simulink model "FloatingBall"  (R2024b)
settings: Solver=FixedStepAuto  StartTime=0.0  StopTime=inf  RelTol=1e-3  EnableMultiTasking=on
undefined symbols (not defined in the file or in its folder): Start
libraries: arduinolib x10, arduinoavrlib x2
(part 1 of 2)
settings Model: ExtModeTrigDuration=2  Creator=Tim  LastModifiedBy=thoma
settings SolverCC: AutoInsertRateTranBlk=on
settings OptimizationCC: DefaultParameterBehavior=Inlined  EnhancedBackFolding=on  PassReuseOutputArgsAs=Individual arguments  ZeroExternalMemoryAtStartup=off  ZeroInternalMemoryAtStartup=off  MaxStackSize=64  OptimizeBlockOrder=speed  DifferentSizesBufferReuse=on  OptimizationCustomize=off  EfficientTunableParamExpr=on
settings DebuggingCC: MultiTaskDSMMsg=none  ParameterTunabilityLossMsg=error
settings HardwareCC: ProdBitPerInt=16  ProdBitPerPointer=16  ProdBitPerSizeT=16  ProdBitPerPtrDiffT=16  ProdLargestAtomicFloat=None  ProdWordSize=8  ProdHWDeviceType=Atmel->AVR
settings SFSimCC: MATLABDynamicMemAlloc=off
settings RTWCC: Description=Embedded Coder  SystemTargetFile=ert.tlc  HardwareBoard=Arduino Uno  TemplateMakefile=ert_default_tmf  Toolchain=Arduino AVR  BuildConfiguration=Faster Runs
settings CodeAppCC: ForceParamTrailComments=on  IgnoreCustomStorageClasses=off  OperatorAnnotations=on  SimulinkDataObjDesc=on  SFDataObjDesc=on  InsertBlockDesc=on
settings ERTTargetCC: SupportContinuousTime=on  SupportVariableSizeSignals=on  ExtModeTransport=3  ExtModeStaticAlloc=on  ExtModeAutomaticAllocSize=off  ExtModeStaticAllocSize=250  ExtModeMexFile=ext_xcp  ExtModeIntrfLevel=Level2 - Open

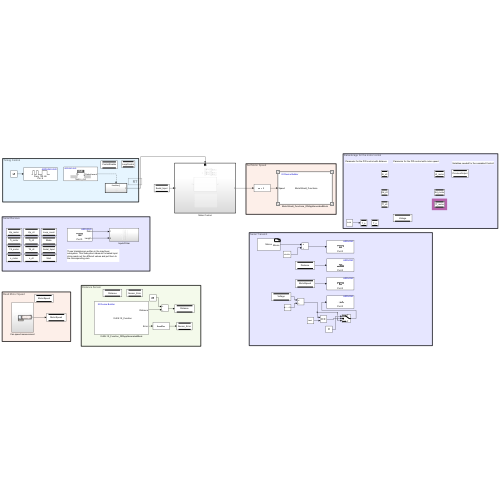
[thumbnail: Simulink's stored preview of the top-level diagram]
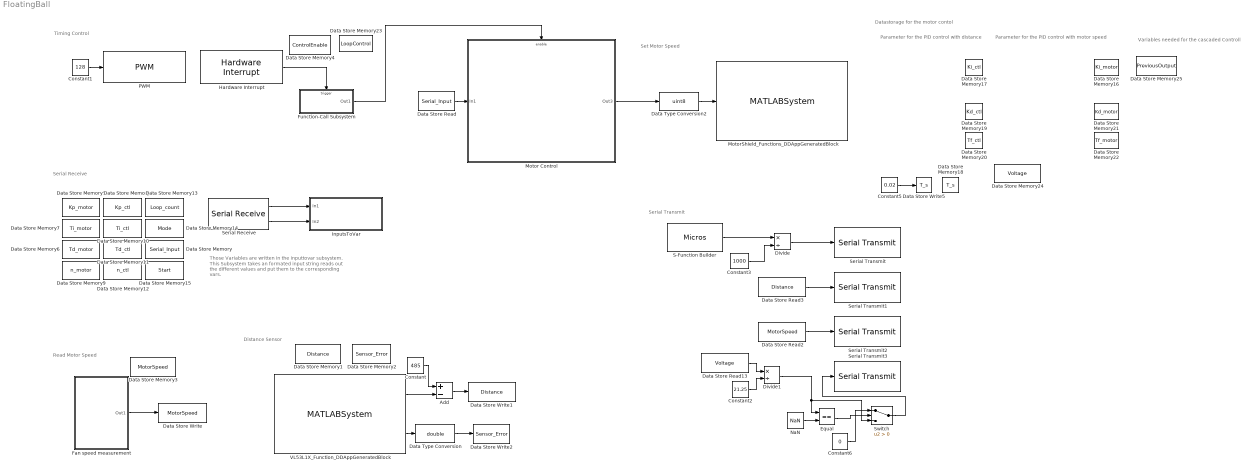
== system FloatingBall ==
  note: Variables needed for the cascaded Controll
  note: Timing Control
  note: Serial Receive
  note: Those Variables are written in the inputtovar subsystem. This Subsystem takes an formated input string reads out the different values and put them to the corresponding vars.
  note: Read Motor Speed
  note: Distance Sensor
  note: Serial Transmit
  note: Set Motor Speed
  note: Parameter for the PID control with distance
  note: Datastorage for the motor contol
  note: Parameter for the PID control with motor speed
  Add : Sum  Inputs=+-
  Constant : Constant  Value=485
  Constant1 : Constant  Value=128
  Constant2 : Constant  Value=21.25
  Constant3 : Constant  Value=1000
  Constant5 : Constant  Value=0.02
  Constant6 : Constant  Value=0
  Data Store Memory : DataStoreMemory  DataStoreName=Serial_Input  WriteAfterWriteMsg=warning  ShowAdditionalParam=off
  Data Store Memory1 : DataStoreMemory  DataStoreName=Distance  WriteAfterWriteMsg=warning  ShowAdditionalParam=off
  Data Store Memory10 : DataStoreMemory  DataStoreName=Ti_ctl  WriteAfterWriteMsg=warning  ShowAdditionalParam=off
  Data Store Memory11 : DataStoreMemory  DataStoreName=Td_ctl  WriteAfterWriteMsg=warning  ShowAdditionalParam=off
  Data Store Memory12 : DataStoreMemory  DataStoreName=n_ctl  WriteAfterWriteMsg=warning  ShowAdditionalParam=off
  Data Store Memory13 : DataStoreMemory  DataStoreName=Loop_count  WriteAfterWriteMsg=warning  ShowAdditionalParam=off
  Data Store Memory14 : DataStoreMemory  DataStoreName=Mode  WriteAfterWriteMsg=warning  ShowAdditionalParam=off
  Data Store Memory15 : DataStoreMemory  DataStoreName=Start  WriteAfterWriteMsg=warning  ShowAdditionalParam=off
  Data Store Memory16 : DataStoreMemory  DataStoreName=Ki_motor  WriteAfterWriteMsg=warning  ShowAdditionalParam=off
  Data Store Memory17 : DataStoreMemory  DataStoreName=Ki_ctl  WriteAfterWriteMsg=warning  ShowAdditionalParam=off
  Data Store Memory18 : DataStoreMemory  DataStoreName=T_s  WriteAfterWriteMsg=warning  ShowAdditionalParam=off
  Data Store Memory19 : DataStoreMemory  DataStoreName=Kd_ctl  WriteAfterWriteMsg=warning  ShowAdditionalParam=off
  Data Store Memory2 : DataStoreMemory  DataStoreName=Sensor_Error  WriteAfterWriteMsg=warning  ShowAdditionalParam=off
  Data Store Memory20 : DataStoreMemory  DataStoreName=Tf_ctl  WriteAfterWriteMsg=warning  ShowAdditionalParam=off
  Data Store Memory21 : DataStoreMemory  DataStoreName=Kd_motor  WriteAfterWriteMsg=warning  ShowAdditionalParam=off
  Data Store Memory22 : DataStoreMemory  DataStoreName=Tf_motor  WriteAfterWriteMsg=warning  ShowAdditionalParam=off
  Data Store Memory23 : DataStoreMemory  DataStoreName=LoopControl  WriteAfterWriteMsg=warning  ShowAdditionalParam=off
  Data Store Memory24 : DataStoreMemory  DataStoreName=Voltage  WriteAfterWriteMsg=warning  ShowAdditionalParam=off
  Data Store Memory25 : DataStoreMemory  DataStoreName=PreviousOutput  WriteAfterWriteMsg=warning  ShowAdditionalParam=off
  Data Store Memory3 : DataStoreMemory  DataStoreName=MotorSpeed  WriteAfterWriteMsg=warning  ShowAdditionalParam=off
  Data Store Memory4 : DataStoreMemory  DataStoreName=ControlEnable  WriteAfterWriteMsg=warning  ShowAdditionalParam=off
  Data Store Memory5 : DataStoreMemory  DataStoreName=Kp_motor  WriteAfterWriteMsg=warning  ShowAdditionalParam=off
  Data Store Memory6 : DataStoreMemory  DataStoreName=Td_motor  WriteAfterWriteMsg=warning  ShowAdditionalParam=off
  Data Store Memory7 : DataStoreMemory  DataStoreName=Ti_motor  WriteAfterWriteMsg=warning  ShowAdditionalParam=off
  Data Store Memory8 : DataStoreMemory  DataStoreName=Kp_ctl  WriteAfterWriteMsg=warning  ShowAdditionalParam=off
  Data Store Memory9 : DataStoreMemory  DataStoreName=n_motor  WriteAfterWriteMsg=warning  ShowAdditionalParam=off
  Data Store Read : DataStoreRead  DataStoreName=Serial_Input  IndexOptions=Index vector (dialog)  Indices=1  OutputSizes=1
  Data Store Read13 : DataStoreRead  DataStoreName=Voltage  IndexOptions=Index vector (dialog)  Indices=1  OutputSizes=1
  Data Store Read2 : DataStoreRead  DataStoreName=MotorSpeed  IndexOptions=Index vector (dialog)  Indices=1  OutputSizes=1
  Data Store Read3 : DataStoreRead  DataStoreName=Distance  IndexOptions=Index vector (dialog)  Indices=1  OutputSizes=1
  Data Store Write : DataStoreWrite  DataStoreName=MotorSpeed  IndexOptions=Index vector (dialog)  Indices=1  OutputSizes=1
  Data Store Write1 : DataStoreWrite  DataStoreName=Distance  IndexOptions=Index vector (dialog)  Indices=1  OutputSizes=1
  Data Store Write2 : DataStoreWrite  DataStoreName=Sensor_Error  IndexOptions=Index vector (dialog)  Indices=1  OutputSizes=1
  Data Store Write5 : DataStoreWrite  DataStoreName=T_s  IndexOptions=Index vector (dialog)  Indices=1  OutputSizes=1
  Data Type Conversion : DataTypeConversion  OutDataTypeStr=double  SaturateOnIntegerOverflow=off  RndMeth=Floor
  Data Type Conversion2 : DataTypeConversion  OutDataTypeStr=uint8  SaturateOnIntegerOverflow=off  RndMeth=Floor
  Divide : Product  Inputs=*/
  Divide1 : Product  Inputs=*/
  Equal : RelationalOperator  Operator===  OutDataTypeStr=boolean  RndMeth=Simplest  InputSameDT=off
  Fan speed measurement : Subsystem
  Function-Call Subsystem : Subsystem  TreatAsAtomicUnit=on
  Hardware Interrupt : arduinoavrlib/Hardware Interrupt  ISRGroup=Timer 1  ISRName=TIMER1_OVF  ISRNumber=7  EventsList={'on','Default event','1'}  SelectedEvents={'Default event'}  TaskPriority=8  DisablePreemption=on  ClearInterruptFlagsAtEndOfEvent=off  HardwareBoard=ARDUINO AVR
  InputsToVar : Subsystem
  Motor Control : Subsystem
  MotorShield_Functions_DDAppGeneratedBlock : MATLABSystem  System=MotorShield_Functions  SampleTime=-1
      mask Type: MotorShield_Functions
      mask Display:
      | color('white');plot([100,100,100,100]*1,[100,100,100,100]*1);plot([100,100,100,100]*0,[100,100,100,100]*0);color('blue');text(38, 92, 'IO Device Builder','horizontalAlignment', 'right');
      | color('black');text(52,50,' MotorShield_Functions','horizontalAlignment','center');
      | port_label('input',1,'Speed');
  NaN : Constant  Value=NaN  OutDataTypeStr=Inherit: Inherit via back propagation
  PWM : arduinoavrlib/PWM  pinNumber=9  desiredFrequency=100  achievableFrequency=100  EnableCompareMatchInterrupt=off  EnableOverflowInterrupt=on
  S-Function Builder : S-Function  FunctionName=Micros  SFunctionModules=Micros_wrapper.c  SFunctionDeploymentMode=off  EnableBusSupport=off  mask(S-Function Builder){}
      mask help: Simulink:masks:SFunctionBuilder_MD
      mask init:
      | val = [[.9  0.75 0.75 1 1 .9 .9 1]',[1 1 0.75 0.75 .9 .9 1 .9]'];try , sys = get_param(gcb,'SfunBuilderFcnName');if isempty(sys), sys = get_param(gcb,'FunctionName'); end,catch, sys = get_param(gcb,'FunctionName'); end
      settings: CopyFcn=set_param(gcbh,'LinkStatus','none')  OpenFcn=sfunctionwizard(gcbh)
      mask Display:
      | plot(val(:,1),val(:,2))
      | disp(sys)
      | port_label('output',1,sprintf('%s', 'Micros'),'interpreter','tex')
  Serial Receive : arduinolib/Serial Receive  portNumber=0  DataType=uint8  blockPlatform=ARDUINO  TimeOut=1000  MaxDataLength=64  isARMArch=off  DataLengthOption=Variable length  Datalength=1  Header=[]  Terminator=[]  SampleTime=0.02  ShowOutStatus=on
  Serial Transmit : arduinolib/Serial Transmit  portNumber=0  sendmode=print  label=;Start:  sendformat=Decimal  floatprecision=2  header=[]  terminator=[]  blockPlatform=ARDUINO
  Serial Transmit1 : arduinolib/Serial Transmit  portNumber=0  sendmode=print  label=;  sendformat=Decimal  floatprecision=1  header=[]  terminator=[]  blockPlatform=ARDUINO
  Serial Transmit2 : arduinolib/Serial Transmit  portNumber=0  sendmode=print  label=;  sendformat=Decimal  floatprecision=1  header=[]  terminator=[]  blockPlatform=ARDUINO
  Serial Transmit3 : arduinolib/Serial Transmit  portNumber=0  sendmode=print  label=;  sendformat=Decimal  floatprecision=2  header=[]  terminator=[]  blockPlatform=ARDUINO
  Switch : Switch  Criteria=u2 > Threshold  SaturateOnIntegerOverflow=off  InputSameDT=off
  VL53L1X_Function_DDAppGeneratedBlock : MATLABSystem  System=VL53L1X_Function  SampleTime=0.02
      mask Type: VL53L1X_Function
      mask Display:
      | color('white');plot([100,100,100,100]*1,[100,100,100,100]*1);plot([100,100,100,100]*0,[100,100,100,100]*0);color('blue');text(38, 92, 'IO Device Builder','horizontalAlignment', 'right');
      | color('black');text(52,50,' VL53L1X_Function','horizontalAlignment','center');
      | port_label('output',1,'Distance');port_label('output',2,'Error');
  wires:
  Constant1/1 -> PWM/1
  Hardware Interrupt/1 -> Function-Call Subsystem/Trigger
  Fan speed measurement/1(Out1) -> Data Store Write/1
  VL53L1X_Function_DDAppGeneratedBlock/2 -> Data Type Conversion/1
  Data Type Conversion/1 -> Data Store Write2/1
  Function-Call Subsystem/1(Out1) -> Motor Control/Enable
  S-Function Builder/1 -> Divide/1
  Constant3/1 -> Divide/2
  Divide/1 -> Serial Transmit/1
  Constant2/1 -> Divide1/2
  Divide1/1 -> Switch/3, Equal/1
  Serial Receive/1 -> InputsToVar/1(In1)
  Serial Receive/2 -> InputsToVar/2(In2)
  Data Store Read/1 -> Motor Control/1(In1)
  Motor Control/1(Out3) -> Data Type Conversion2/1
  Data Type Conversion2/1 -> MotorShield_Functions_DDAppGeneratedBlock/1
  Constant5/1 -> Data Store Write5/1
  Add/1 -> Data Store Write1/1
  Constant/1 -> Add/1
  VL53L1X_Function_DDAppGeneratedBlock/1 -> Add/2
  Data Store Read13/1 -> Divide1/1
  NaN/1 -> Equal/2
  Equal/1 -> Switch/2
  Switch/1 -> Serial Transmit3/1
  Constant6/1 -> Switch/1
  Data Store Read2/1 -> Serial Transmit2/1
  Data Store Read3/1 -> Serial Transmit1/1

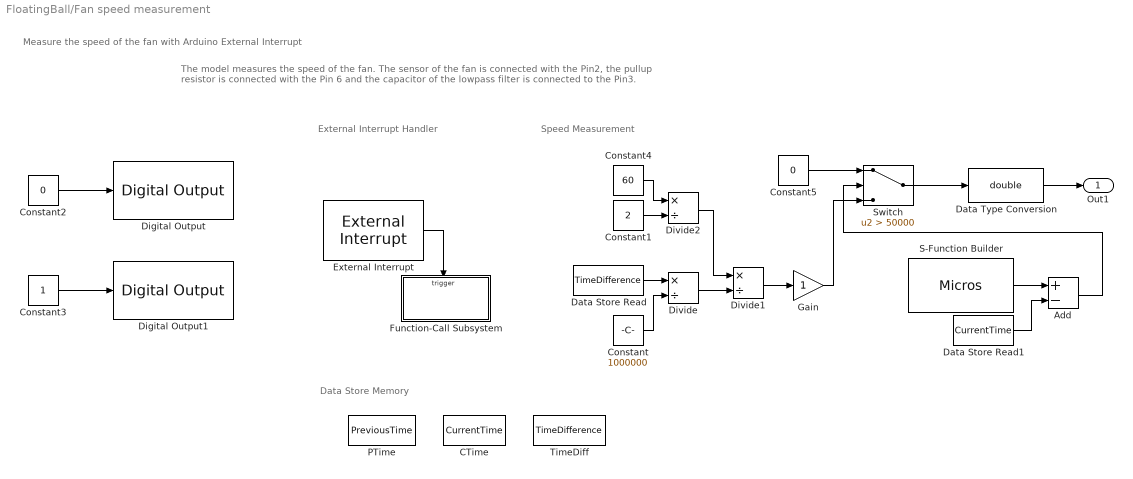
== system FloatingBall/Fan speed measurement ==
  note: External Interrupt Handler
  note: Speed Measurement
  note: Data Store Memory
  note: Measure the speed of the fan with Arduino External Interrupt
  note: The model measures the speed of the fan.
      | The sensor of the fan is connected with the Pin2, the pullup resistor is connected with the Pin 6 and
      | the capacitor of the lowpass filter is connected to the Pin3.
  Add : Sum  Inputs=+-
  CTime : DataStoreMemory  DataStoreName=CurrentTime  ShowAdditionalParam=off  OutDataTypeStr=uint32
  Constant : Constant  Value=1000000
  Constant1 : Constant  Value=2
  Constant2 : Constant  Value=0
  Constant3 : Constant
  Constant4 : Constant  Value=60
  Constant5 : Constant  Value=0
  Data Store Read : DataStoreRead  DataStoreName=TimeDifference  IndexOptions=Index vector (dialog)  Indices=1  OutputSizes=1
  Data Store Read1 : DataStoreRead  DataStoreName=CurrentTime  IndexOptions=Index vector (dialog)  Indices=1  OutputSizes=1
  Data Type Conversion : DataTypeConversion  OutDataTypeStr=double  SaturateOnIntegerOverflow=off  RndMeth=Floor
  Digital Output : arduinolib/Digital Output  pinNumber=3  Direction=output  blockPlatform=arduino
  Digital Output1 : arduinolib/Digital Output  pinNumber=6  Direction=output  blockPlatform=arduino
  Divide : Product  Inputs=*/
  Divide1 : Product  Inputs=*/
  Divide2 : Product  Inputs=*/
  External Interrupt : arduinolib/External Interrupt  Pin=2  PullUp=off  Mode=FALLING  InterruptSimulationInput=off
  Function-Call Subsystem : Subsystem  TreatAsAtomicUnit=on
  Gain : Gain
  PTime : DataStoreMemory  DataStoreName=PreviousTime  ShowAdditionalParam=off  OutDataTypeStr=uint32
  S-Function Builder : S-Function  FunctionName=Micros  SFunctionModules=Micros_wrapper.c  SFunctionDeploymentMode=off  EnableBusSupport=off  mask(S-Function Builder){}
      mask help: Simulink:masks:SFunctionBuilder_MD
      mask init: same as FloatingBall/S-Function Builder
      settings: CopyFcn=set_param(gcbh,'LinkStatus','none')  OpenFcn=sfunctionwizard(gcbh)
      mask Display:
      | plot(val(:,1),val(:,2))
      | disp(sys)
      | port_label('output',1,sprintf('%s', 'Micros'),'interpreter','tex')
  Switch : Switch  Criteria=u2 > Threshold  Threshold=50000  SaturateOnIntegerOverflow=off  InputSameDT=off
  TimeDiff : DataStoreMemory  DataStoreName=TimeDifference  ShowAdditionalParam=off  OutDataTypeStr=uint32
  Out1 : Outport
  wires:
  Divide/1 -> Divide1/2
  Constant/1 -> Divide/2
  External Interrupt/1 -> Function-Call Subsystem/Trigger
  Constant1/1 -> Divide2/2
  Data Store Read/1 -> Divide/1
  Constant3/1 -> Digital Output1/1
  Constant2/1 -> Digital Output/1
  Constant4/1 -> Divide2/1
  Data Type Conversion/1 -> Out1/1
  Divide2/1 -> Divide1/1
  Divide1/1 -> Gain/1
  S-Function Builder/1 -> Add/1
  Data Store Read1/1 -> Add/2
  Add/1 -> Switch/2
  Switch/1 -> Data Type Conversion/1
  Gain/1 -> Switch/3
  Constant5/1 -> Switch/1

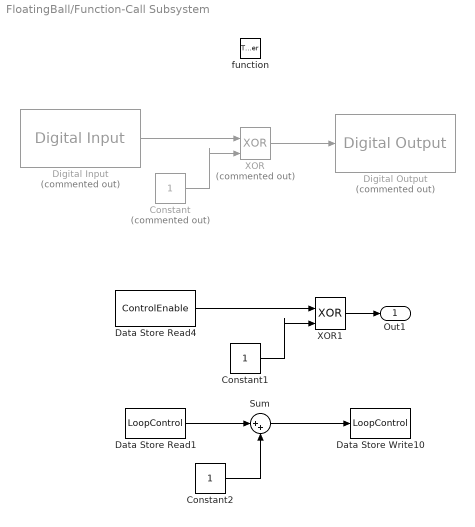
== system FloatingBall/Function-Call Subsystem ==
  function : TriggerPort  TriggerType=function-call  VariantControl=(inherit)
  Constant : Constant  Commented=on
  Constant1 : Constant
  Constant2 : Constant
  Data Store Read1 : DataStoreRead  DataStoreName=LoopControl  IndexOptions=Index vector (dialog)  Indices=1  OutputSizes=1
  Data Store Read4 : DataStoreRead  DataStoreName=ControlEnable  IndexOptions=Index vector (dialog)  Indices=1  OutputSizes=1
  Data Store Write10 : DataStoreWrite  DataStoreName=LoopControl  IndexOptions=Index vector (dialog)  Indices=1  OutputSizes=1
  Digital Input : arduinolib/Digital Input  Commented=on  pinNumber=12  mode=Default  Direction=input  SampleTime=-1  blockPlatform=arduino
  Digital Output : arduinolib/Digital Output  Commented=on  pinNumber=13  Direction=output  blockPlatform=arduino
  Sum : Sum  Inputs=|++
  XOR : Logic  Commented=on  Operator=XOR  IconShape=distinctive  AllPortsSameDT=off  OutDataTypeStr=boolean
  XOR1 : Logic  Operator=XOR  IconShape=distinctive  AllPortsSameDT=off  OutDataTypeStr=boolean
  Out1 : Outport
  wires:
  Constant/1 -> XOR/2
  Digital Input/1 -> XOR/1
  XOR/1 -> Digital Output/1
  Constant1/1 -> XOR1/2
  Data Store Read4/1 -> XOR1/1
  XOR1/1 -> Out1/1
  Data Store Read1/1 -> Sum/1
  Sum/1 -> Data Store Write10/1
  Constant2/1 -> Sum/2

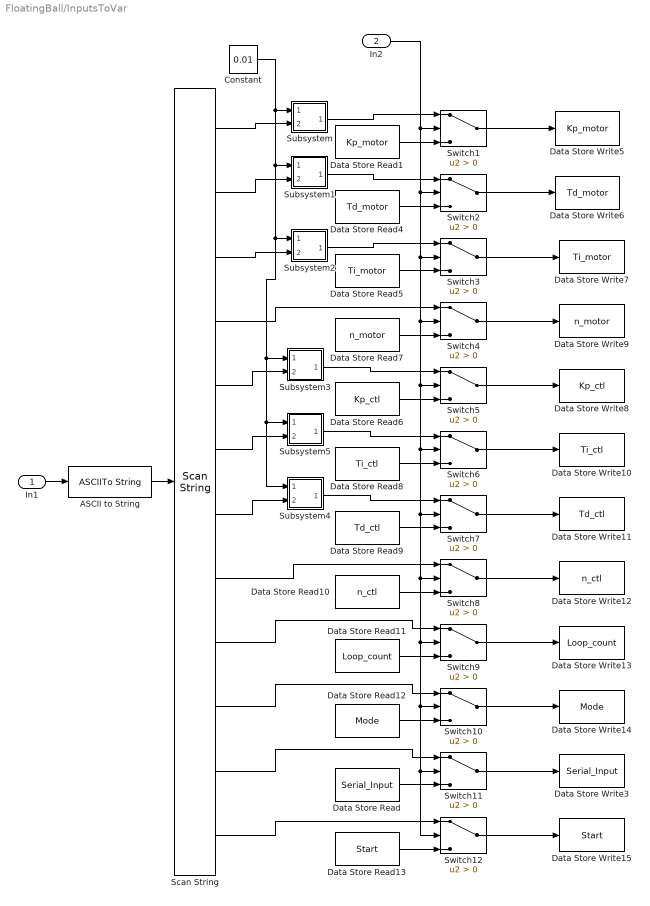
== system FloatingBall/InputsToVar ==
  In1 : Inport
  In2 : Inport  Port=2
  ASCII to String : ASCIIToString
  Constant : Constant  Value=0.01
  Data Store Read : DataStoreRead  DataStoreName=Serial_Input  IndexOptions=Index vector (dialog)  Indices=1  OutputSizes=1
  Data Store Read1 : DataStoreRead  DataStoreName=Kp_motor  IndexOptions=Index vector (dialog)  Indices=1  OutputSizes=1
  Data Store Read10 : DataStoreRead  DataStoreName=n_ctl  IndexOptions=Index vector (dialog)  Indices=1  OutputSizes=1
  Data Store Read11 : DataStoreRead  DataStoreName=Loop_count  IndexOptions=Index vector (dialog)  Indices=1  OutputSizes=1
  Data Store Read12 : DataStoreRead  DataStoreName=Mode  IndexOptions=Index vector (dialog)  Indices=1  OutputSizes=1
  Data Store Read13 : DataStoreRead  DataStoreName=Start  IndexOptions=Index vector (dialog)  Indices=1  OutputSizes=1
  Data Store Read4 : DataStoreRead  DataStoreName=Td_motor  IndexOptions=Index vector (dialog)  Indices=1  OutputSizes=1
  Data Store Read5 : DataStoreRead  DataStoreName=Ti_motor  IndexOptions=Index vector (dialog)  Indices=1  OutputSizes=1
  Data Store Read6 : DataStoreRead  DataStoreName=Kp_ctl  IndexOptions=Index vector (dialog)  Indices=1  OutputSizes=1
  Data Store Read7 : DataStoreRead  DataStoreName=n_motor  IndexOptions=Index vector (dialog)  Indices=1  OutputSizes=1
  Data Store Read8 : DataStoreRead  DataStoreName=Ti_ctl  IndexOptions=Index vector (dialog)  Indices=1  OutputSizes=1
  Data Store Read9 : DataStoreRead  DataStoreName=Td_ctl  IndexOptions=Index vector (dialog)  Indices=1  OutputSizes=1
  Data Store Write10 : DataStoreWrite  DataStoreName=Ti_ctl  IndexOptions=Index vector (dialog)  Indices=1  OutputSizes=1
  Data Store Write11 : DataStoreWrite  DataStoreName=Td_ctl  IndexOptions=Index vector (dialog)  Indices=1  OutputSizes=1
  Data Store Write12 : DataStoreWrite  DataStoreName=n_ctl  IndexOptions=Index vector (dialog)  Indices=1  OutputSizes=1
  Data Store Write13 : DataStoreWrite  DataStoreName=Loop_count  IndexOptions=Index vector (dialog)  Indices=1  OutputSizes=1
  Data Store Write14 : DataStoreWrite  DataStoreName=Mode  IndexOptions=Index vector (dialog)  Indices=1  OutputSizes=1
  Data Store Write15 : DataStoreWrite  DataStoreName=Start  IndexOptions=Index vector (dialog)  Indices=1  OutputSizes=1
  Data Store Write3 : DataStoreWrite  DataStoreName=Serial_Input  IndexOptions=Index vector (dialog)  Indices=1  OutputSizes=1
  Data Store Write5 : DataStoreWrite  DataStoreName=Kp_motor  IndexOptions=Index vector (dialog)  Indices=1  OutputSizes=1
  Data Store Write6 : DataStoreWrite  DataStoreName=Td_motor  IndexOptions=Index vector (dialog)  Indices=1  OutputSizes=1
  Data Store Write7 : DataStoreWrite  DataStoreName=Ti_motor  IndexOptions=Index vector (dialog)  Indices=1  OutputSizes=1
  Data Store Write8 : DataStoreWrite  DataStoreName=Kp_ctl  IndexOptions=Index vector (dialog)  Indices=1  OutputSizes=1
  Data Store Write9 : DataStoreWrite  DataStoreName=n_motor  IndexOptions=Index vector (dialog)  Indices=1  OutputSizes=1
  Scan String : ScanString  Format="\"%d %d %d %d %d %d %d %d %d %d %d %d\""
  Subsystem : Subsystem
  Subsystem1 : Subsystem
  Subsystem2 : Subsystem
  Subsystem3 : Subsystem
  Subsystem4 : Subsystem
  Subsystem5 : Subsystem
  Switch{1..12} (12 alike) : Switch  Criteria=u2 > Threshold  SaturateOnIntegerOverflow=off  InputSameDT=off
  wires:
  ASCII to String/1 -> Scan String/1
  In1/1 -> ASCII to String/1
  Data Store Read1/1 -> Switch1/3
  Data Store Read4/1 -> Switch2/3
  Switch2/1 -> Data Store Write6/1
  In2/1 -> Switch1/2, Switch2/2, Switch3/2, Switch4/2, Switch5/2, Switch12/2, Switch11/2, Switch10/2, Switch9/2, Switch8/2, Switch7/2, Switch6/2
  Data Store Read5/1 -> Switch3/3
  Switch3/1 -> Data Store Write7/1
  Data Store Read11/1 -> Switch9/3
  Switch9/1 -> Data Store Write13/1
  Switch8/1 -> Data Store Write12/1
  Data Store Read10/1 -> Switch8/3
  Data Store Read9/1 -> Switch7/3
  Switch7/1 -> Data Store Write11/1
  Data Store Read12/1 -> Switch10/3
  Data Store Read/1 -> Switch11/3
  Data Store Read13/1 -> Switch12/3
  Switch12/1 -> Data Store Write15/1
  Switch11/1 -> Data Store Write3/1
  Switch6/1 -> Data Store Write10/1
  Data Store Read8/1 -> Switch6/3
  Data Store Read6/1 -> Switch5/3
  Switch5/1 -> Data Store Write8/1
  Data Store Read7/1 -> Switch4/3
  Switch4/1 -> Data Store Write9/1
  Scan String/1 -> Subsystem/2(In1)
  Scan String/2 -> Subsystem1/2(In1)
  Scan String/3 -> Subsystem2/2(In1)
  Scan String/4 -> Switch4/1
  Scan String/5 -> Subsystem3/2(In1)
  Scan String/6 -> Subsystem5/2(In1)
  Scan String/7 -> Subsystem4/2(In1)
  Scan String/8 -> Switch8/1
  Scan String/9 -> Switch9/1
  Scan String/10 -> Switch10/1
  Scan String/11 -> Switch11/1
  Scan String/12 -> Switch12/1
  Switch1/1 -> Data Store Write5/1
  Subsystem1/1(Out1) -> Switch2/1
  Subsystem/1(Out1) -> Switch1/1
  Subsystem2/1(Out1) -> Switch3/1
  Subsystem3/1(Out1) -> Switch5/1
  Subsystem5/1(Out1) -> Switch6/1
  Subsystem4/1(Out1) -> Switch7/1
  Switch10/1 -> Data Store Write14/1
  Constant/1 -> Subsystem1/1(In2), Subsystem2/1(In2), Subsystem3/1(In2), Subsystem4/1(In2), Subsystem5/1(In2), Subsystem/1(In2)

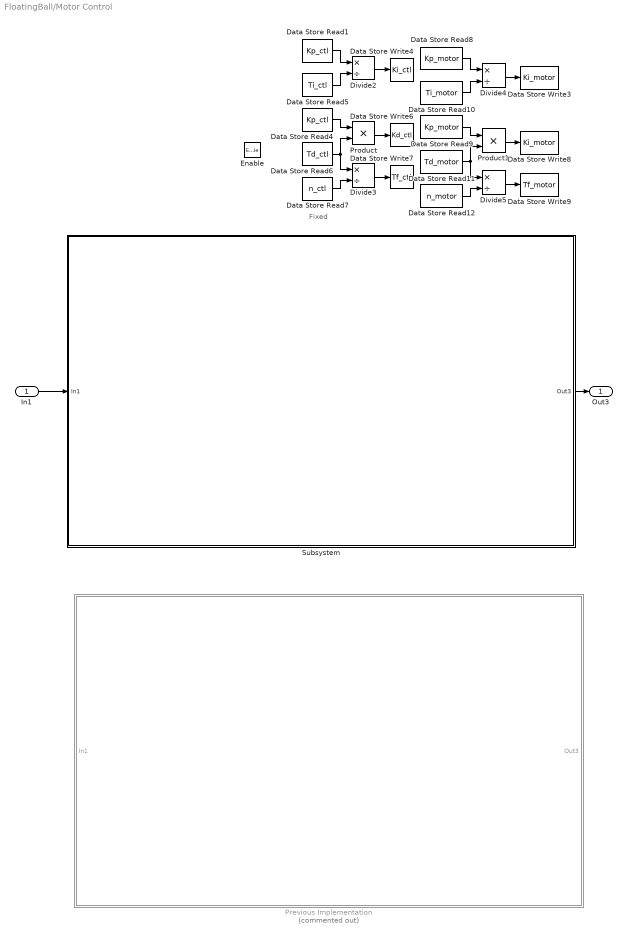
== system FloatingBall/Motor Control ==
  note: Fixed
  In1 : Inport
  Enable : EnablePort
  Data Store Read1 : DataStoreRead  DataStoreName=Kp_ctl  IndexOptions=Index vector (dialog)  Indices=1  OutputSizes=1
  Data Store Read10 : DataStoreRead  DataStoreName=Ti_motor  IndexOptions=Index vector (dialog)  Indices=1  OutputSizes=1
  Data Store Read11 : DataStoreRead  DataStoreName=Td_motor  IndexOptions=Index vector (dialog)  Indices=1  OutputSizes=1
  Data Store Read12 : DataStoreRead  DataStoreName=n_motor  IndexOptions=Index vector (dialog)  Indices=1  OutputSizes=1
  Data Store Read4 : DataStoreRead  DataStoreName=Kp_ctl  IndexOptions=Index vector (dialog)  Indices=1  OutputSizes=1
  Data Store Read5 : DataStoreRead  DataStoreName=Ti_ctl  IndexOptions=Index vector (dialog)  Indices=1  OutputSizes=1
  Data Store Read6 : DataStoreRead  DataStoreName=Td_ctl  IndexOptions=Index vector (dialog)  Indices=1  OutputSizes=1
  Data Store Read7 : DataStoreRead  DataStoreName=n_ctl  IndexOptions=Index vector (dialog)  Indices=1  OutputSizes=1
  Data Store Read8 : DataStoreRead  DataStoreName=Kp_motor  IndexOptions=Index vector (dialog)  Indices=1  OutputSizes=1
  Data Store Read9 : DataStoreRead  DataStoreName=Kp_motor  IndexOptions=Index vector (dialog)  Indices=1  OutputSizes=1
  Data Store Write3 : DataStoreWrite  DataStoreName=Ki_motor  IndexOptions=Index vector (dialog)  Indices=1  OutputSizes=1
  Data Store Write4 : DataStoreWrite  DataStoreName=Ki_ctl  IndexOptions=Index vector (dialog)  Indices=1  OutputSizes=1
  Data Store Write6 : DataStoreWrite  DataStoreName=Kd_ctl  IndexOptions=Index vector (dialog)  Indices=1  OutputSizes=1
  Data Store Write7 : DataStoreWrite  DataStoreName=Tf_ctl  IndexOptions=Index vector (dialog)  Indices=1  OutputSizes=1
  Data Store Write8 : DataStoreWrite  DataStoreName=Ki_motor  IndexOptions=Index vector (dialog)  Indices=1  OutputSizes=1
  Data Store Write9 : DataStoreWrite  DataStoreName=Tf_motor  IndexOptions=Index vector (dialog)  Indices=1  OutputSizes=1
  Divide{2..5} (4 alike) : Product  Inputs=*/
  Previous Implementation : Subsystem  Commented=on
  Product : Product
  Product1 : Product
  Subsystem : Subsystem
  Out3 : Outport
  wires:
  In1/1 -> Subsystem/1(In1)
  Subsystem/1(Out3) -> Out3/1
  Divide3/1 -> Data Store Write7/1
  Product/1 -> Data Store Write6/1
  Data Store Read4/1 -> Product/1
  Data Store Read11/1 -> Divide5/1, Product1/2
  Data Store Read8/1 -> Divide4/1
  Data Store Read7/1 -> Divide3/2
  Divide4/1 -> Data Store Write3/1
  Data Store Read6/1 -> Divide3/1, Product/2
  Product1/1 -> Data Store Write8/1
  Divide5/1 -> Data Store Write9/1
  Data Store Read5/1 -> Divide2/2
  Divide2/1 -> Data Store Write4/1
  Data Store Read10/1 -> Divide4/2
  Data Store Read1/1 -> Divide2/1
  Data Store Read9/1 -> Product1/1
  Data Store Read12/1 -> Divide5/2

== system FloatingBall/Fan speed measurement/Function-Call Subsystem ==
  isr_handler : TriggerPort  TriggerType=function-call  VariantControl=Variant
  Data Store Read : DataStoreRead  DataStoreName=CurrentTime  IndexOptions=Index vector (dialog)  Indices=1  OutputSizes=1
  Data Store Read1 : DataStoreRead  DataStoreName=PreviousTime  IndexOptions=Index vector (dialog)  Indices=1  OutputSizes=1
  Data Store Read2 : DataStoreRead  DataStoreName=CurrentTime  IndexOptions=Index vector (dialog)  Indices=1  OutputSizes=1
  Data Store Write : DataStoreWrite  Priority=1  DataStoreName=CurrentTime  IndexOptions=Index vector (dialog)  Indices=1  OutputSizes=1
  Data Store Write1 : DataStoreWrite  Priority=2  DataStoreName=TimeDifference  IndexOptions=Index vector (dialog)  Indices=1  OutputSizes=1
  Data Store Write2 : DataStoreWrite  Priority=3  DataStoreName=PreviousTime  IndexOptions=Index vector (dialog)  Indices=1  OutputSizes=1
  S-Function Builder : S-Function  FunctionName=Micros  SFunctionModules=Micros_wrapper.c  SFunctionDeploymentMode=off  EnableBusSupport=off  mask(S-Function Builder){}
      mask help: Simulink:masks:SFunctionBuilder_MD
      mask init: same as FloatingBall/S-Function Builder
      settings: CopyFcn=set_param(gcbh,'LinkStatus','none')  OpenFcn=sfunctionwizard(gcbh)
      mask Display:
      | plot(val(:,1),val(:,2))
      | disp(sys)
      | port_label('output',1,sprintf('%s', 'Micros'),'interpreter','tex')
  Subtract : Sum  Inputs=+-
  wires:
  S-Function Builder/1 -> Data Store Write/1
  Data Store Read/1 -> Subtract/1
  Data Store Read1/1 -> Subtract/2
  Subtract/1 -> Data Store Write1/1
  Data Store Read2/1 -> Data Store Write2/1

== system FloatingBall/InputsToVar/Subsystem ==
  In2 : Inport
  In1 : Inport  Port=2
  Cast To Double : DataTypeConversion  OutDataTypeStr=double  SaturateOnIntegerOverflow=off  RndMeth=Floor
  Product : Product
  Out1 : Outport
  wires:
  Cast To Double/1 -> Product/2
  Product/1 -> Out1/1
  In1/1 -> Cast To Double/1
  In2/1 -> Product/1

== system FloatingBall/InputsToVar/Subsystem1 ==
  In2 : Inport
  In1 : Inport  Port=2
  Cast To Double : DataTypeConversion  OutDataTypeStr=double  SaturateOnIntegerOverflow=off  RndMeth=Floor
  Product : Product
  Out1 : Outport
  wires:
  Product/1 -> Out1/1
  In1/1 -> Cast To Double/1
  Cast To Double/1 -> Product/2
  In2/1 -> Product/1

== system FloatingBall/InputsToVar/Subsystem2 ==
  In2 : Inport
  In1 : Inport  Port=2
  Cast To Double : DataTypeConversion  OutDataTypeStr=double  SaturateOnIntegerOverflow=off  RndMeth=Floor
  Product : Product
  Out1 : Outport
  wires:
  Product/1 -> Out1/1
  In1/1 -> Cast To Double/1
  Cast To Double/1 -> Product/2
  In2/1 -> Product/1

== system FloatingBall/InputsToVar/Subsystem3 ==
  In2 : Inport
  In1 : Inport  Port=2
  Cast To Double : DataTypeConversion  OutDataTypeStr=double  SaturateOnIntegerOverflow=off  RndMeth=Floor
  Product : Product
  Out1 : Outport
  wires:
  Product/1 -> Out1/1
  In1/1 -> Cast To Double/1
  Cast To Double/1 -> Product/2
  In2/1 -> Product/1

== system FloatingBall/InputsToVar/Subsystem4 ==
  In2 : Inport
  In1 : Inport  Port=2
  Cast To Double : DataTypeConversion  OutDataTypeStr=double  SaturateOnIntegerOverflow=off  RndMeth=Floor
  Product : Product
  Out1 : Outport
  wires:
  Product/1 -> Out1/1
  In1/1 -> Cast To Double/1
  Cast To Double/1 -> Product/2
  In2/1 -> Product/1

== system FloatingBall/InputsToVar/Subsystem5 ==
  In2 : Inport
  In1 : Inport  Port=2
  Cast To Double : DataTypeConversion  OutDataTypeStr=double  SaturateOnIntegerOverflow=off  RndMeth=Floor
  Product : Product
  Out1 : Outport
  wires:
  Product/1 -> Out1/1
  In1/1 -> Cast To Double/1
  Cast To Double/1 -> Product/2
  In2/1 -> Product/1

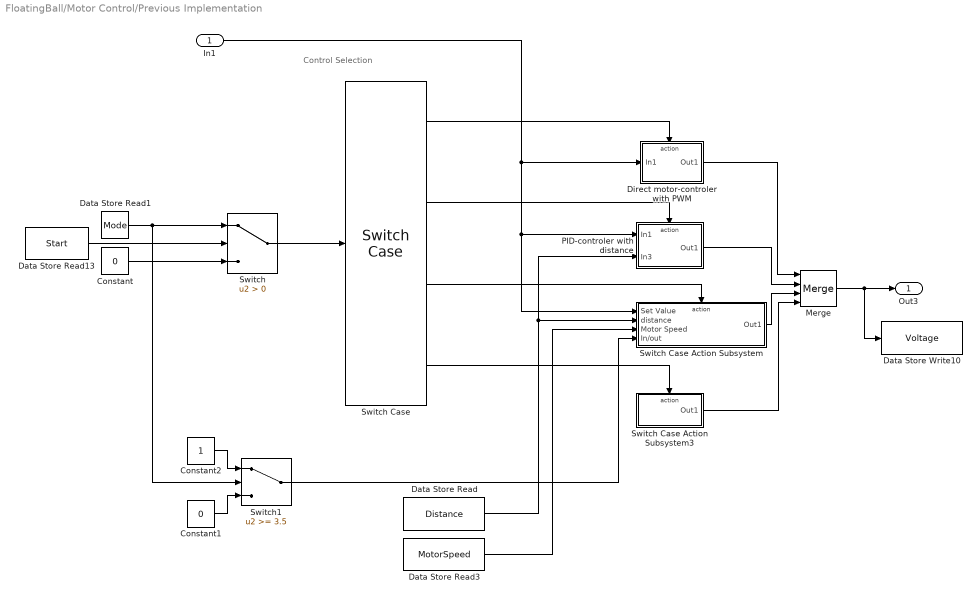
== system FloatingBall/Motor Control/Previous Implementation ==
  note: Control Selection
  In1 : Inport
  Constant : Constant  Value=0
  Constant1 : Constant  Value=0
  Constant2 : Constant
  Data Store Read : DataStoreRead  DataStoreName=Distance  IndexOptions=Index vector (dialog)  Indices=1  OutputSizes=1
  Data Store Read1 : DataStoreRead  DataStoreName=Mode  IndexOptions=Index vector (dialog)  Indices=1  OutputSizes=1
  Data Store Read13 : DataStoreRead  DataStoreName=Start  IndexOptions=Index vector (dialog)  Indices=1  OutputSizes=1
  Data Store Read3 : DataStoreRead  DataStoreName=MotorSpeed  IndexOptions=Index vector (dialog)  Indices=1  OutputSizes=1
  Data Store Write10 : DataStoreWrite  DataStoreName=Voltage  IndexOptions=Index vector (dialog)  Indices=1  OutputSizes=1
  Direct motor-controler with PWM : Subsystem  TreatAsAtomicUnit=on
  Merge : Merge  Inputs=4
  PID-controler with distance : Subsystem  TreatAsAtomicUnit=on
  Switch : Switch  Criteria=u2 > Threshold  SaturateOnIntegerOverflow=off  InputSameDT=off
  Switch Case : SwitchCase  CaseConditions={1,2,[3,4]}
  Switch Case Action Subsystem : Subsystem  TreatAsAtomicUnit=on
  Switch Case Action Subsystem3 : Subsystem  TreatAsAtomicUnit=on
  Switch1 : Switch  Threshold=3.5  SaturateOnIntegerOverflow=off  InputSameDT=off
  Out3 : Outport
  wires:
  Switch Case/4 -> Switch Case Action Subsystem3/Action
  Data Store Read/1 -> Switch Case Action Subsystem/2(distance), PID-controler with distance/2(In3)
  In1/1 -> Direct motor-controler with PWM/1(In1), Switch Case Action Subsystem/1(Set Value), PID-controler with distance/1(In1)
  Switch Case/3 -> Switch Case Action Subsystem/Action
  Switch Case/2 -> PID-controler with distance/Action
  Switch Case/1 -> Direct motor-controler with PWM/Action
  Switch/1 -> Switch Case/1
  Data Store Read3/1 -> Switch Case Action Subsystem/3(Motor Speed)
  Merge/1 -> Data Store Write10/1, Out3/1
  Switch Case Action Subsystem3/1(Out1) -> Merge/4
  Direct motor-controler with PWM/1(Out1) -> Merge/1
  PID-controler with distance/1(Out1) -> Merge/2
  Switch Case Action Subsystem/1(Out1) -> Merge/3
  Data Store Read13/1 -> Switch/2
  Data Store Read1/1 -> Switch1/2, Switch/1
  Constant/1 -> Switch/3
  Constant1/1 -> Switch1/3
  Constant2/1 -> Switch1/1
  Switch1/1 -> Switch Case Action Subsystem/4(In/out)

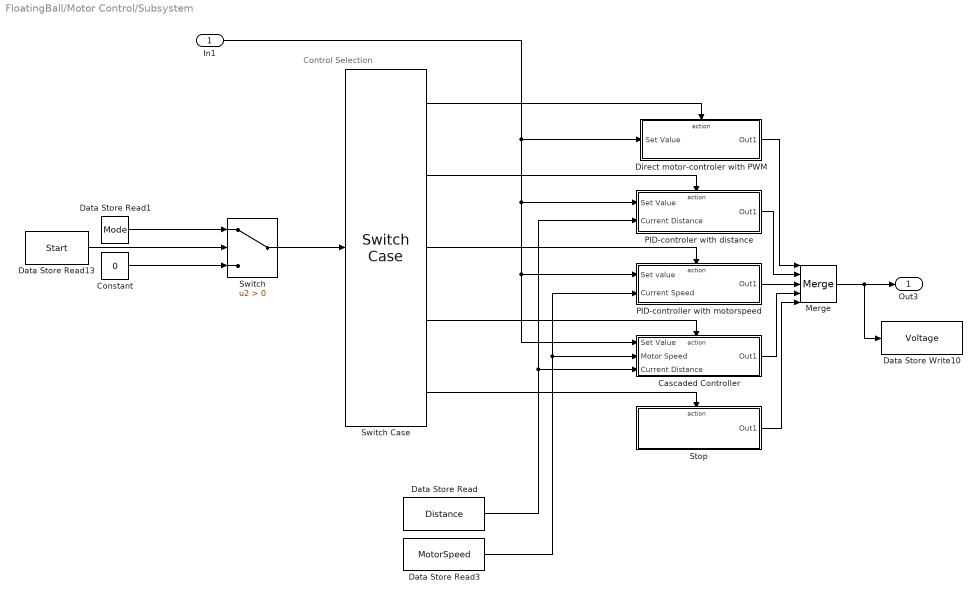
== system FloatingBall/Motor Control/Subsystem ==
  note: Control Selection
  In1 : Inport
  Cascaded Controller : Subsystem  TreatAsAtomicUnit=on
  Constant : Constant  Value=0
  Data Store Read : DataStoreRead  DataStoreName=Distance  IndexOptions=Index vector (dialog)  Indices=1  OutputSizes=1
  Data Store Read1 : DataStoreRead  DataStoreName=Mode  IndexOptions=Index vector (dialog)  Indices=1  OutputSizes=1
  Data Store Read13 : DataStoreRead  DataStoreName=Start  IndexOptions=Index vector (dialog)  Indices=1  OutputSizes=1
  Data Store Read3 : DataStoreRead  DataStoreName=MotorSpeed  IndexOptions=Index vector (dialog)  Indices=1  OutputSizes=1
  Data Store Write10 : DataStoreWrite  DataStoreName=Voltage  IndexOptions=Index vector (dialog)  Indices=1  OutputSizes=1
  Direct motor-controler with PWM : Subsystem  TreatAsAtomicUnit=on
  Merge : Merge  Inputs=5  InitialOutput=[0]
  PID-controler with distance : Subsystem  TreatAsAtomicUnit=on
  PID-controller with motorspeed : Subsystem  TreatAsAtomicUnit=on
  Stop : Subsystem  TreatAsAtomicUnit=on
  Switch : Switch  Criteria=u2 > Threshold  SaturateOnIntegerOverflow=off  InputSameDT=off
  Switch Case : SwitchCase  CaseConditions={1,2,3,4}
  Out3 : Outport
  wires:
  Switch Case/5 -> Stop/Action
  Data Store Read/1 -> PID-controler with distance/2(Current Distance), Cascaded Controller/3(Current Distance)
  In1/1 -> Cascaded Controller/1(Set Value), PID-controller with motorspeed/1(Set value), PID-controler with distance/1(Set Value), Direct motor-controler with PWM/1(Set Value)
  Switch Case/3 -> PID-controller with motorspeed/Action
  Switch Case/2 -> PID-controler with distance/Action
  Switch Case/1 -> Direct motor-controler with PWM/Action
  Switch/1 -> Switch Case/1
  Data Store Read3/1 -> PID-controller with motorspeed/2(Current Speed), Cascaded Controller/2(Motor Speed)
  Merge/1 -> Data Store Write10/1, Out3/1
  Stop/1(Out1) -> Merge/5
  Direct motor-controler with PWM/1(Out1) -> Merge/1
  PID-controler with distance/1(Out1) -> Merge/2
  PID-controller with motorspeed/1(Out1) -> Merge/3
  Data Store Read13/1 -> Switch/2
  Data Store Read1/1 -> Switch/1
  Constant/1 -> Switch/3
  Switch Case/4 -> Cascaded Controller/Action
  Cascaded Controller/1(Out1) -> Merge/4

== system FloatingBall/Motor Control/Previous Implementation/Direct motor-controler with PWM ==
  In1 : Inport
  Action Port : ActionPort
  Gain : Gain  Gain="255   /   3200"
  Out1 : Outport
  wires:
  In1/1 -> Gain/1
  Gain/1 -> Out1/1

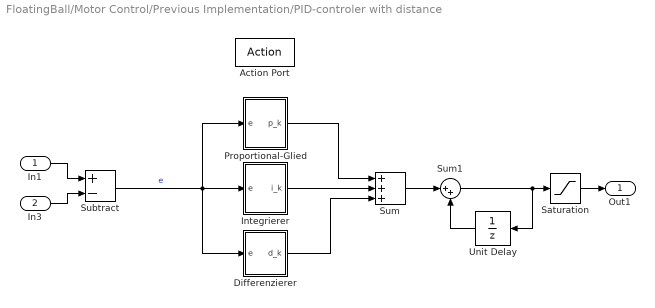
== system FloatingBall/Motor Control/Previous Implementation/PID-controler with distance ==
  In1 : Inport
  In3 : Inport  Port=2
  Action Port : ActionPort
  Differenzierer : Subsystem
  Integrierer : Subsystem
  Proportional-Glied : Subsystem
  Saturation : Saturate  UpperLimit=255  LowerLimit=0
  Subtract : Sum  Inputs=+-
  Sum : Sum  Inputs=+++
  Sum1 : Sum  Inputs=|++
  Unit Delay : UnitDelay  SampleTime=0.02  HasFrameUpgradeWarning=on
  Out1 : Outport
  wires:
  Sum/1 -> Sum1/1
  Integrierer/1(i_k) -> Sum/2
  Proportional-Glied/1(p_k) -> Sum/1
  Differenzierer/1(d_k) -> Sum/3
  Subtract/1 -> Integrierer/1(e), Differenzierer/1(e), Proportional-Glied/1(e)  "e"
  In1/1 -> Subtract/1
  In3/1 -> Subtract/2
  Saturation/1 -> Out1/1
  Sum1/1 -> Unit Delay/1, Saturation/1
  Unit Delay/1 -> Sum1/2

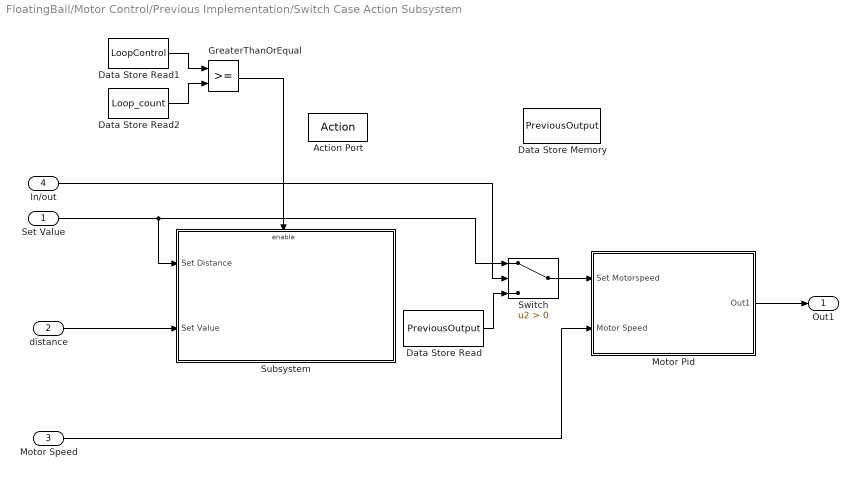
== system FloatingBall/Motor Control/Previous Implementation/Switch Case Action Subsystem ==
  Set Value : Inport
  distance : Inport  Port=2
  Motor Speed : Inport  Port=3
  In/out : Inport  Port=4
  Action Port : ActionPort
  Data Store Memory : DataStoreMemory  DataStoreName=PreviousOutput  WriteAfterWriteMsg=warning  ShowAdditionalParam=off
  Data Store Read : DataStoreRead  DataStoreName=PreviousOutput  IndexOptions=Index vector (dialog)  Indices=1  OutputSizes=1
  Data Store Read1 : DataStoreRead  DataStoreName=LoopControl  IndexOptions=Index vector (dialog)  Indices=1  OutputSizes=1
  Data Store Read2 : DataStoreRead  DataStoreName=Loop_count  IndexOptions=Index vector (dialog)  Indices=1  OutputSizes=1
  GreaterThanOrEqual : RelationalOperator  OutDataTypeStr=boolean  RndMeth=Simplest  InputSameDT=off
  Motor Pid : Subsystem
  Subsystem : Subsystem
  Switch : Switch  Criteria=u2 > Threshold  SaturateOnIntegerOverflow=off  InputSameDT=off
  Out1 : Outport
  wires:
  Motor Pid/1(Out1) -> Out1/1
  Motor Speed/1 -> Motor Pid/2(Motor Speed)
  Set Value/1 -> Subsystem/1(Set Distance), Switch/1
  In/out/1 -> Switch/2
  Switch/1 -> Motor Pid/1(Set Motorspeed)
  Data Store Read/1 -> Switch/3
  distance/1 -> Subsystem/2(Set Value)
  Data Store Read2/1 -> GreaterThanOrEqual/2
  Data Store Read1/1 -> GreaterThanOrEqual/1
  GreaterThanOrEqual/1 -> Subsystem/Enable

== system FloatingBall/Motor Control/Previous Implementation/Switch Case Action Subsystem3 ==
  Action Port : ActionPort
  Constant : Constant  Value=0
  Out1 : Outport
  wires:
  Constant/1 -> Out1/1

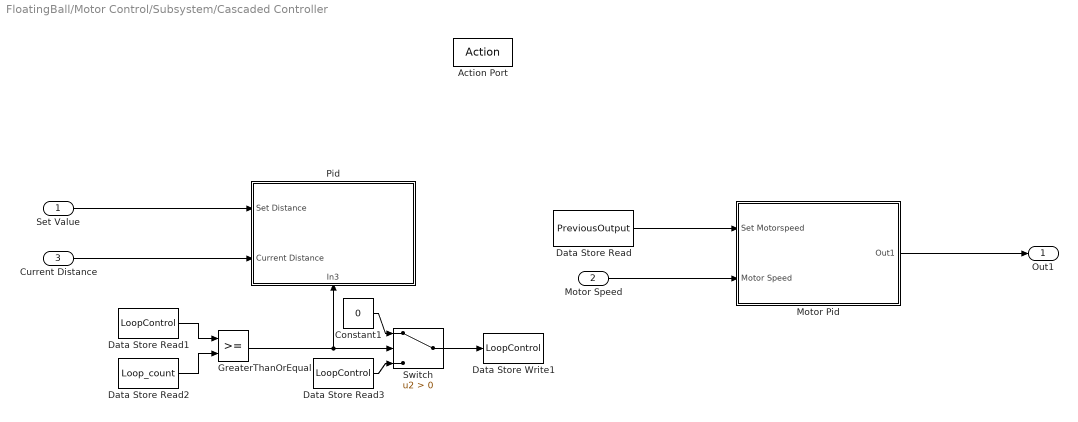
== system FloatingBall/Motor Control/Subsystem/Cascaded Controller ==
  Set Value : Inport
  Motor Speed : Inport  Port=2
  Current Distance : Inport  Port=3
  Action Port : ActionPort  ActionPortLabel=case [ 4 ]:
  Constant1 : Constant  Value=0
  Data Store Read : DataStoreRead  DataStoreName=PreviousOutput  IndexOptions=Index vector (dialog)  Indices=1  OutputSizes=1
  Data Store Read1 : DataStoreRead  DataStoreName=LoopControl  IndexOptions=Index vector (dialog)  Indices=1  OutputSizes=1
  Data Store Read2 : DataStoreRead  DataStoreName=Loop_count  IndexOptions=Index vector (dialog)  Indices=1  OutputSizes=1
  Data Store Read3 : DataStoreRead  DataStoreName=LoopControl  IndexOptions=Index vector (dialog)  Indices=1  OutputSizes=1
  Data Store Write1 : DataStoreWrite  DataStoreName=LoopControl  IndexOptions=Index vector (dialog)  Indices=1  OutputSizes=1
  GreaterThanOrEqual : RelationalOperator  OutDataTypeStr=boolean  RndMeth=Simplest  InputSameDT=off
  Motor Pid : Subsystem
  Pid : Subsystem
      settings: PortSchema="{\"entries\":[{\"content\":{\"sides\":[{\"content\":{\"connectorIds\":[\"In1\",\"In2\"]},\"type\":\"ConnectorPlacement.EquallySpacedRectSide\",\"uuid\":\"6ad93547-b11d-4498-bf86-2badffcf62b4\"},{\"content\":{\"side\":\"RIGHT\"},\"type\":\"ConnectorPlacement.EquallySpacedRectSide\",\"uuid\":\"b91d1434-0ca6-4c9b-8aeb-b62dfb2b5798\"},{\"content\":{\"side\":\"TOP\"},\"type\":\"ConnectorPlacement.EquallySpacedRectSide\",\"uuid\":\"db87fbcb-9053-460a-a1a1-3f5de7359bda\"},{\"content\":{\"connectorIds\":[\"In3\"],\"side\":\"BOTTOM\"},\"type\":\"ConnectorPlacement.EquallySpacedRectSide\",\"uuid\":\"cfa2024b-2b7d-4817-875c-c191708dfdf1\"}]},\"type\":\"ConnectorPlacement.EquallySpacedConnector\",\"uuid\":\"4a39c175-8512-41b5-b57d-1a8985d3d7a8\"}],\"packageUris\":[\"http://schema.mathworks.com/mf0/Connector/R2020b\"],\"version\":\"1.0\"}"
  Switch : Switch  Criteria=u2 > Threshold  SaturateOnIntegerOverflow=off  InputSameDT=off
  Out1 : Outport
  wires:
  Motor Pid/1(Out1) -> Out1/1
  Data Store Read1/1 -> GreaterThanOrEqual/1
  GreaterThanOrEqual/1 -> Switch/2, Pid/3(In3)
  Data Store Read2/1 -> GreaterThanOrEqual/2
  Set Value/1 -> Pid/1(Set Distance)
  Current Distance/1 -> Pid/2(Current Distance)
  Motor Speed/1 -> Motor Pid/2(Motor Speed)
  Data Store Read/1 -> Motor Pid/1(Set Motorspeed)
  Constant1/1 -> Switch/1
  Switch/1 -> Data Store Write1/1
  Data Store Read3/1 -> Switch/3

== system FloatingBall/Motor Control/Subsystem/Direct motor-controler with PWM ==
  Set Value : Inport
  Action Port : ActionPort  ActionPortLabel=case [ 1 ]:
  Cast To Double : DataTypeConversion  OutDataTypeStr=double  SaturateOnIntegerOverflow=off  RndMeth=Floor
  Gain : Gain  Gain="255   /   3200"
  Out1 : Outport
  wires:
  Set Value/1 -> Cast To Double/1
  Gain/1 -> Out1/1
  Cast To Double/1 -> Gain/1

== system FloatingBall/Motor Control/Subsystem/PID-controler with distance ==
  Set Value : Inport
  Current Distance : Inport  Port=2
  Action Port : ActionPort  ActionPortLabel=case [ 2 ]:
  Differenzierer : Subsystem
  Integrierer : Subsystem
  Proportional-Glied : Subsystem
  Saturation : Saturate  UpperLimit=255  LowerLimit=0
  Subtract : Sum  Inputs=+-
  Sum : Sum  Inputs=+++
  Sum1 : Sum  Inputs=|++
  Unit Delay : UnitDelay  SampleTime=0.02  HasFrameUpgradeWarning=on
  Out1 : Outport
  wires:
  Sum/1 -> Sum1/1
  Integrierer/1(i_k) -> Sum/2
  Proportional-Glied/1(p_k) -> Sum/1
  Differenzierer/1(d_k) -> Sum/3
  Subtract/1 -> Integrierer/1(e), Differenzierer/1(e), Proportional-Glied/1(e)  "e"
  Set Value/1 -> Subtract/1
  Current Distance/1 -> Subtract/2
  Saturation/1 -> Out1/1
  Sum1/1 -> Unit Delay/1, Saturation/1
  Unit Delay/1 -> Sum1/2

== system FloatingBall/Motor Control/Subsystem/PID-controller with motorspeed ==
  Set value : Inport
  Current Speed : Inport  Port=2
  Action Port : ActionPort  ActionPortLabel=case [ 3 ]:
  Differenzierer : Subsystem
  Integrierer : Subsystem
  Proportional-Glied : Subsystem
  Saturation : Saturate  UpperLimit=255  LowerLimit=0
  Subtract : Sum  Inputs=+-
  Sum : Sum  Inputs=+++
  Sum1 : Sum  Inputs=|++
  Unit Delay : UnitDelay  SampleTime=0.02  HasFrameUpgradeWarning=on
  Out1 : Outport
  wires:
  Sum1/1 -> Unit Delay/1, Saturation/1
  Differenzierer/1(d_k) -> Sum/3
  Proportional-Glied/1(p_k) -> Sum/1
  Unit Delay/1 -> Sum1/2
  Set value/1 -> Subtract/1
  Subtract/1 -> Integrierer/1(e), Differenzierer/1(e), Proportional-Glied/1(e)  "e"
  Saturation/1 -> Out1/1
  Current Speed/1 -> Subtract/2
  Sum/1 -> Sum1/1
  Integrierer/1(i_k) -> Sum/2

== system FloatingBall/Motor Control/Subsystem/Stop ==
  Action Port : ActionPort  ActionPortLabel=default:
  Constant : Constant  Value=0
  Out1 : Outport
  wires:
  Constant/1 -> Out1/1

== system FloatingBall/Motor Control/Previous Implementation/PID-controler with distance/Differenzierer ==
  e : Inport
  Add : Sum
  Data Store Read : DataStoreRead  DataStoreName=Tf_motor  IndexOptions=Index vector (dialog)  Indices=1  OutputSizes=1
  Data Store Read1 : DataStoreRead  DataStoreName=T_s  IndexOptions=Index vector (dialog)  Indices=1  OutputSizes=1
  Data Store Read2 : DataStoreRead  DataStoreName=Kd_motor  IndexOptions=Index vector (dialog)  Indices=1  OutputSizes=1
  Divide : Product  Inputs=**/
  Divide1 : Product  Inputs=**/
  Sum : Sum  Inputs=|+-
  Sum1 : Sum  Inputs=|++
  Unit Delay : UnitDelay  SampleTime=0.02  HasFrameUpgradeWarning=on
  Unit Delay1 : UnitDelay  SampleTime=0.02  HasFrameUpgradeWarning=on
  d_k : Outport
  wires:
  Sum1/1 -> Unit Delay1/1, d_k/1  "d_k"
  Divide/1 -> Sum1/1
  e/1 -> Unit Delay/1, Sum/1
  Sum/1 -> Divide/2
  Unit Delay/1 -> Sum/2
  Divide1/1 -> Sum1/2
  Unit Delay1/1 -> Divide1/1  "d_k-1"
  Add/1 -> Divide1/3, Divide/3
  Data Store Read1/1 -> Add/1
  Data Store Read/1 -> Divide1/2, Add/2
  Data Store Read2/1 -> Divide/1

== system FloatingBall/Motor Control/Previous Implementation/PID-controler with distance/Integrierer ==
  e : Inport
  Constant : Constant  Value=2
  Data Store Read : DataStoreRead  DataStoreName=Ki_motor  IndexOptions=Index vector (dialog)  Indices=1  OutputSizes=1
  Data Store Read1 : DataStoreRead  DataStoreName=T_s  IndexOptions=Index vector (dialog)  Indices=1  OutputSizes=1
  Divide : Product  Inputs=***/
  Sum : Sum  Inputs=|++
  Sum1 : Sum  Inputs=|++
  Unit Delay : UnitDelay  SampleTime=0.02  HasFrameUpgradeWarning=on
  Unit Delay1 : UnitDelay  SampleTime=0.02  HasFrameUpgradeWarning=on
  i_k : Outport
  wires:
  Divide/1 -> Unit Delay1/1, Sum1/1
  Sum/1 -> Divide/2
  e/1 -> Sum/1, Unit Delay/1
  Sum1/1 -> i_k/1
  Unit Delay1/1 -> Sum1/2
  Data Store Read1/1 -> Divide/3
  Unit Delay/1 -> Sum/2
  Data Store Read/1 -> Divide/1
  Constant/1 -> Divide/4

== system FloatingBall/Motor Control/Previous Implementation/PID-controler with distance/Proportional-Glied ==
  e : Inport
  Data Store Read : DataStoreRead  DataStoreName=Kp_motor  IndexOptions=Index vector (dialog)  Indices=1  OutputSizes=1
  Product : Product
  p_k : Outport
  wires:
  Product/1 -> p_k/1  "p_k"
  e/1 -> Product/2
  Data Store Read/1 -> Product/1

== system FloatingBall/Motor Control/Previous Implementation/Switch Case Action Subsystem/Motor Pid ==
  Set Motorspeed : Inport
  Motor Speed : Inport  Port=2
  Differenzierer : Subsystem
  Integrierer : Subsystem
  Proportional-Glied : Subsystem
  Saturation : Saturate  UpperLimit=255  LowerLimit=0
  Subtract : Sum  Inputs=+-
  Sum : Sum  Inputs=+++
  Sum1 : Sum  Inputs=|++
  Unit Delay : UnitDelay  SampleTime=0.02  HasFrameUpgradeWarning=on
  Out1 : Outport
  wires:
  Integrierer/1(i_k) -> Sum/2
  Unit Delay/1 -> Sum1/2
  Sum1/1 -> Unit Delay/1, Saturation/1
  Proportional-Glied/1(p_k) -> Sum/1
  Set Motorspeed/1 -> Subtract/1
  Sum/1 -> Sum1/1
  Subtract/1 -> Integrierer/1(e), Differenzierer/1(e), Proportional-Glied/1(e)  "e"
  Differenzierer/1(d_k) -> Sum/3
  Saturation/1 -> Out1/1
  Motor Speed/1 -> Subtract/2

== system FloatingBall/Motor Control/Previous Implementation/Switch Case Action Subsystem/Subsystem ==
  Set Distance : Inport
  Set Value : Inport  Port=2
  Enable : EnablePort
  Pid : Subsystem
  wires:
  Set Value/1 -> Pid/2(Set Value)
  Set Distance/1 -> Pid/1(Set Distance)

== system FloatingBall/Motor Control/Subsystem/Cascaded Controller/Motor Pid ==
  Set Motorspeed : Inport
  Motor Speed : Inport  Port=2
  Differenzierer : Subsystem
  Integrierer : Subsystem
  Proportional-Glied : Subsystem
  Saturation : Saturate  UpperLimit=255  LowerLimit=0
  Subtract : Sum  Inputs=+-
  Sum : Sum  Inputs=+++
  Sum1 : Sum  Inputs=|++
  Unit Delay : UnitDelay  SampleTime=0.02  HasFrameUpgradeWarning=on
  Out1 : Outport
  wires:
  Integrierer/1(i_k) -> Sum/2
  Unit Delay/1 -> Sum1/2
  Sum1/1 -> Unit Delay/1, Saturation/1
  Proportional-Glied/1(p_k) -> Sum/1
  Set Motorspeed/1 -> Subtract/1
  Sum/1 -> Sum1/1
  Subtract/1 -> Integrierer/1(e), Differenzierer/1(e), Proportional-Glied/1(e)  "e"
  Differenzierer/1(d_k) -> Sum/3
  Saturation/1 -> Out1/1
  Motor Speed/1 -> Subtract/2

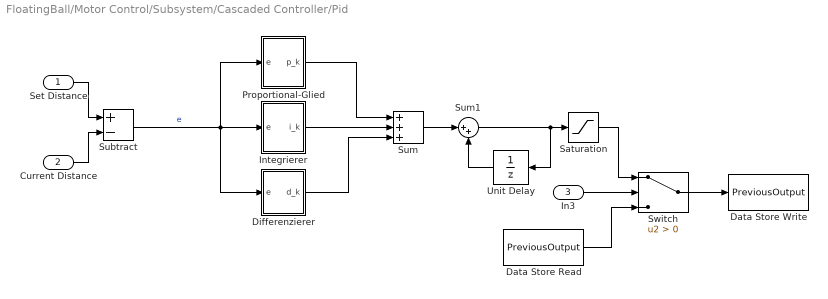
== system FloatingBall/Motor Control/Subsystem/Cascaded Controller/Pid ==
  Set Distance : Inport
  Current Distance : Inport  Port=2
  In3 : Inport  Port=3
  Data Store Read : DataStoreRead  DataStoreName=PreviousOutput  IndexOptions=Index vector (dialog)  Indices=1  OutputSizes=1
  Data Store Write : DataStoreWrite  DataStoreName=PreviousOutput  IndexOptions=Index vector (dialog)  Indices=1  OutputSizes=1
  Differenzierer : Subsystem
  Integrierer : Subsystem
  Proportional-Glied : Subsystem
  Saturation : Saturate  UpperLimit=3100  LowerLimit=0
  Subtract : Sum  Inputs=+-
  Sum : Sum  Inputs=+++
  Sum1 : Sum  Inputs=|++
  Switch : Switch  Criteria=u2 > Threshold  SaturateOnIntegerOverflow=off  InputSameDT=off
  Unit Delay : UnitDelay  SampleTime=0.02  HasFrameUpgradeWarning=on
  wires:
  Integrierer/1(i_k) -> Sum/2
  Unit Delay/1 -> Sum1/2
  Sum1/1 -> Unit Delay/1, Saturation/1
  Proportional-Glied/1(p_k) -> Sum/1
  Current Distance/1 -> Subtract/2
  Sum/1 -> Sum1/1
  Subtract/1 -> Integrierer/1(e), Differenzierer/1(e), Proportional-Glied/1(e)  "e"
  Differenzierer/1(d_k) -> Sum/3
  Saturation/1 -> Switch/1
  Set Distance/1 -> Subtract/1
  In3/1 -> Switch/2
  Switch/1 -> Data Store Write/1
  Data Store Read/1 -> Switch/3

== system FloatingBall/Motor Control/Subsystem/PID-controler with distance/Differenzierer ==
  e : Inport
  Add : Sum
  Data Store Read : DataStoreRead  DataStoreName=Tf_motor  IndexOptions=Index vector (dialog)  Indices=1  OutputSizes=1
  Data Store Read1 : DataStoreRead  DataStoreName=T_s  IndexOptions=Index vector (dialog)  Indices=1  OutputSizes=1
  Data Store Read2 : DataStoreRead  DataStoreName=Kd_motor  IndexOptions=Index vector (dialog)  Indices=1  OutputSizes=1
  Divide : Product  Inputs=**/
  Divide1 : Product  Inputs=**/
  Sum : Sum  Inputs=|+-
  Sum1 : Sum  Inputs=|++
  Unit Delay : UnitDelay  SampleTime=0.02  HasFrameUpgradeWarning=on
  Unit Delay1 : UnitDelay  SampleTime=0.02  HasFrameUpgradeWarning=on
  d_k : Outport
  wires:
  Sum1/1 -> Unit Delay1/1, d_k/1  "d_k"
  Divide/1 -> Sum1/1
  e/1 -> Unit Delay/1, Sum/1
  Sum/1 -> Divide/2
  Unit Delay/1 -> Sum/2
  Divide1/1 -> Sum1/2
  Unit Delay1/1 -> Divide1/1  "d_k-1"
  Add/1 -> Divide1/3, Divide/3
  Data Store Read1/1 -> Add/1
  Data Store Read/1 -> Divide1/2, Add/2
  Data Store Read2/1 -> Divide/1

== system FloatingBall/Motor Control/Subsystem/PID-controler with distance/Integrierer ==
  e : Inport
  Constant : Constant  Value=2
  Data Store Read : DataStoreRead  DataStoreName=Ki_motor  IndexOptions=Index vector (dialog)  Indices=1  OutputSizes=1
  Data Store Read1 : DataStoreRead  DataStoreName=T_s  IndexOptions=Index vector (dialog)  Indices=1  OutputSizes=1
  Divide : Product  Inputs=***/
  Sum : Sum  Inputs=|++
  Sum1 : Sum  Inputs=|++
  Unit Delay : UnitDelay  SampleTime=0.02  HasFrameUpgradeWarning=on
  Unit Delay1 : UnitDelay  SampleTime=0.02  HasFrameUpgradeWarning=on
  i_k : Outport
  wires:
  Divide/1 -> Unit Delay1/1, Sum1/1
  Sum/1 -> Divide/2
  e/1 -> Sum/1, Unit Delay/1
  Sum1/1 -> i_k/1
  Unit Delay1/1 -> Sum1/2
  Data Store Read1/1 -> Divide/3
  Unit Delay/1 -> Sum/2
  Data Store Read/1 -> Divide/1
  Constant/1 -> Divide/4

== system FloatingBall/Motor Control/Subsystem/PID-controler with distance/Proportional-Glied ==
  e : Inport
  Data Store Read : DataStoreRead  DataStoreName=Kp_motor  IndexOptions=Index vector (dialog)  Indices=1  OutputSizes=1
  Product : Product
  p_k : Outport
  wires:
  Product/1 -> p_k/1  "p_k"
  e/1 -> Product/2
  Data Store Read/1 -> Product/1

== system FloatingBall/Motor Control/Subsystem/PID-controller with motorspeed/Differenzierer ==
  e : Inport
  Add : Sum
  Data Store Read : DataStoreRead  DataStoreName=Tf_motor  IndexOptions=Index vector (dialog)  Indices=1  OutputSizes=1
  Data Store Read1 : DataStoreRead  DataStoreName=T_s  IndexOptions=Index vector (dialog)  Indices=1  OutputSizes=1
  Data Store Read2 : DataStoreRead  DataStoreName=Kd_motor  IndexOptions=Index vector (dialog)  Indices=1  OutputSizes=1
  Divide : Product  Inputs=**/
  Divide1 : Product  Inputs=**/
  Sum : Sum  Inputs=|+-
  Sum1 : Sum  Inputs=|++
  Unit Delay : UnitDelay  SampleTime=0.02  HasFrameUpgradeWarning=on
  Unit Delay1 : UnitDelay  SampleTime=0.02  HasFrameUpgradeWarning=on
  d_k : Outport
  wires:
  Sum1/1 -> Unit Delay1/1, d_k/1  "d_k"
  Divide/1 -> Sum1/1
  e/1 -> Unit Delay/1, Sum/1
  Sum/1 -> Divide/2
  Unit Delay/1 -> Sum/2
  Divide1/1 -> Sum1/2
  Unit Delay1/1 -> Divide1/1  "d_k-1"
  Add/1 -> Divide1/3, Divide/3
  Data Store Read1/1 -> Add/1
  Data Store Read/1 -> Divide1/2, Add/2
  Data Store Read2/1 -> Divide/1

== system FloatingBall/Motor Control/Subsystem/PID-controller with motorspeed/Integrierer ==
  e : Inport
  Constant : Constant  Value=2
  Data Store Read : DataStoreRead  DataStoreName=Ki_motor  IndexOptions=Index vector (dialog)  Indices=1  OutputSizes=1
  Data Store Read1 : DataStoreRead  DataStoreName=T_s  IndexOptions=Index vector (dialog)  Indices=1  OutputSizes=1
  Divide : Product  Inputs=***/
  Sum : Sum  Inputs=|++
  Sum1 : Sum  Inputs=|++
  Unit Delay : UnitDelay  SampleTime=0.02  HasFrameUpgradeWarning=on
  Unit Delay1 : UnitDelay  SampleTime=0.02  HasFrameUpgradeWarning=on
  i_k : Outport
  wires:
  Divide/1 -> Unit Delay1/1, Sum1/1
  Sum/1 -> Divide/2
  e/1 -> Sum/1, Unit Delay/1
  Sum1/1 -> i_k/1
  Unit Delay1/1 -> Sum1/2
  Data Store Read1/1 -> Divide/3
  Unit Delay/1 -> Sum/2
  Data Store Read/1 -> Divide/1
  Constant/1 -> Divide/4

== system FloatingBall/Motor Control/Subsystem/PID-controller with motorspeed/Proportional-Glied ==
  e : Inport
  Data Store Read : DataStoreRead  DataStoreName=Kp_motor  IndexOptions=Index vector (dialog)  Indices=1  OutputSizes=1
  Product : Product
  p_k : Outport
  wires:
  Product/1 -> p_k/1  "p_k"
  e/1 -> Product/2
  Data Store Read/1 -> Product/1
